simulink model "scara_controller"  (Simulink 8.1)
settings: Solver=ode1  SolverMode=SingleTasking  StartTime=0.0  StopTime=inf  RelTol=1e-3
PreLoadFcn:
  | waijung.modelPreload; % Required for working with Waijung Blockset. Do not remove.
undefined symbols (not defined in the file or in its folder): ARM, disable_customio, enable_customio, in1, in2, Link, LQFP100, MDK, out1, out2, out3, out4, out5, out6, output_customio, ST, STM32F407VG, STM32F4DISCOVERY
libraries: simulink x6, stm32f4_io_lib x3, USBVCP_STM32F4 x2, waijung_customcode x1, stm32f4_adc_lib x1, stm32f4_device_config_lib x1
(part 2 of 2)

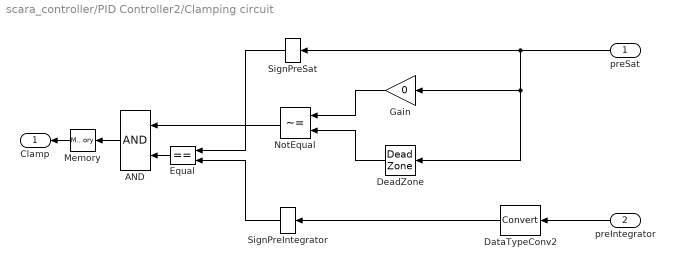
== system scara_controller/PID Controller2/Clamping circuit ==
  preSat : Inport
  preIntegrator : Inport  Port=2
  AND : Logic  DisableCoverage=on  OutDataTypeStr=boolean
  DataTypeConv2 : DataTypeConversion  DisableCoverage=on
  DeadZone : DeadZone  DisableCoverage=on  LowerValue=LowerSaturationLimit  UpperValue=UpperSaturationLimit
  Equal : RelationalOperator  DisableCoverage=on  Operator===  OutDataTypeStr=boolean
  Gain : Gain  DisableCoverage=on  Gain=0  SaturateOnIntegerOverflow=on  OutDataTypeStr=Inherit: Same as input  ParamDataTypeStr=Inherit: Same as input
  Memory : Memory  DisableCoverage=on
  NotEqual : RelationalOperator  DisableCoverage=on  Operator=~=  OutDataTypeStr=boolean
  SignPreIntegrator : Signum  DisableCoverage=on
  SignPreSat : Signum  DisableCoverage=on
  Clamp : Outport
  wires:
  preSat/1 -> DeadZone/1, Gain/1, SignPreSat/1
  preIntegrator/1 -> DataTypeConv2/1
  DataTypeConv2/1 -> SignPreIntegrator/1
  Gain/1 -> NotEqual/1
  DeadZone/1 -> NotEqual/2
  SignPreSat/1 -> Equal/1
  NotEqual/1 -> AND/1
  SignPreIntegrator/1 -> Equal/2
  Equal/1 -> AND/2
  AND/1 -> Memory/1
  Memory/1 -> Clamp/1
